simulink model "Suspension_System"  (R2020b)
settings: Solver=VariableStepAuto  StartTime=0.0  StopTime=100  RelTol=1e-3
PreLoadFcn:
  | clearvars
  | load('Data.mat')
undefined symbols (not defined in the file): b, k1, k2, m1, m2
settings Model: Creator=vigne  LastModifiedBy=prabhudevmaddipudi

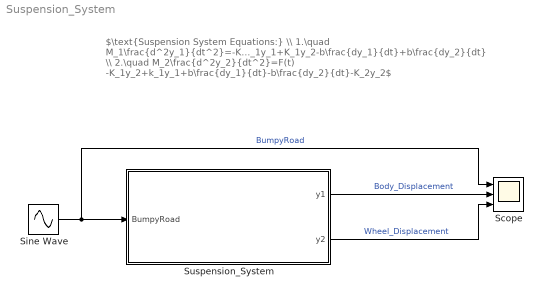
== system Suspension_System ==
  note: $\text{Suspension System Equations:} \\ 1.\quad M_1\frac{d^2y_1}{dt^2}=-K_1y_1+K_1y_2-b\frac{dy_1}{dt}+b\frac{dy_2}{dt} \\ 2.\quad M_2\frac{d^2y_2}{dt^2}=F(t) -K_1y_2+k_1y_1+b\frac{dy_1}{dt}-b\frac{dy_2}{dt}-K_2y_2$
  Scope : Scope  NumInputPorts=3
  Sine Wave : Sin  SampleTime=0
  Suspension_System : Subsystem
  wires:
  Sine Wave/1 -> Scope/1, Suspension_System/1(BumpyRoad)  "BumpyRoad"
  Suspension_System/1(y1) -> Scope/2  "Body_Displacement"
  Suspension_System/2(y2) -> Scope/3  "Wheel_Displacement"

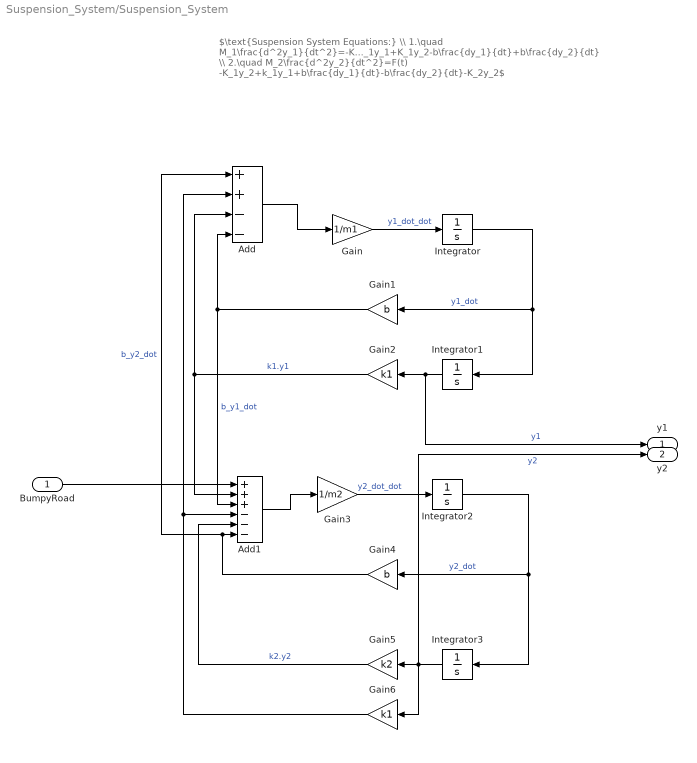
== system Suspension_System/Suspension_System ==
  note: $\text{Suspension System Equations:} \\ 1.\quad M_1\frac{d^2y_1}{dt^2}=-K_1y_1+K_1y_2-b\frac{dy_1}{dt}+b\frac{dy_2}{dt} \\ 2.\quad M_2\frac{d^2y_2}{dt^2}=F(t) -K_1y_2+k_1y_1+b\frac{dy_1}{dt}-b\frac{dy_2}{dt}-K_2y_2$
  BumpyRoad : Inport
  Add : Sum  Inputs=++--
  Add1 : Sum  Inputs=+++---
  Gain : Gain  Gain=1/m1
  Gain1 : Gain  Gain=b
  Gain2 : Gain  Gain=k1
  Gain3 : Gain  Gain=1/m2
  Gain4 : Gain  Gain=b
  Gain5 : Gain  Gain=k2
  Gain6 : Gain  Gain=k1
  Integrator{,1..3} (4 alike) : Integrator
  y1 : Outport
  y2 : Outport  Port=2
  wires:
  Integrator/1 -> Integrator1/1, Gain1/1  "y1_dot"
  Gain5/1 -> Add1/5  "k2.y2"
  Add/1 -> Gain/1
  Gain/1 -> Integrator/1  "y1_dot_dot"
  Gain1/1 -> Add/4, Add1/3  "b_y1_dot"
  Gain4/1 -> Add/1, Add1/6  "b_y2_dot"
  Add1/1 -> Gain3/1
  Integrator2/1 -> Integrator3/1, Gain4/1  "y2_dot"
  Integrator1/1 -> y1/1, Gain2/1  "y1"
  Gain2/1 -> Add1/2, Add/3  "k1.y1"
  Gain6/1 -> Add/2, Add1/4
  Gain3/1 -> Integrator2/1  "y2_dot_dot"
  Integrator3/1 -> y2/1, Gain6/1, Gain5/1  "y2"
  BumpyRoad/1 -> Add1/1
